simulink library "aerolib6dof2"  (Simulink 6.0)
settings: Solver=ode45  SolverMode=SingleTasking  StartTime=0.0  StopTime=10.0  RelTol=1e-3
values from neighbouring files (symbols this model uses):
  s = aeroliblist    [asbhelp.m]
undefined symbols (not defined in the file or in its folder): m
libraries: aerolib6dof2 x5, aerolib6dofsys x2, aerolibutil x2, aerolibconvert x2, simulink x1
settings Model: Creator=sgage  LastModifiedBy=sgage  ExtModeAutoUpdateStatusClock=off
settings DataIOCC: SignalLoggingName=logsOut
settings OptimizationCC: BooleanDataType=off
settings DebuggingCC: CheckExecutionContextPreStartOutputMsg=on  CheckExecutionContextRuntimeOutputMsg=on  SolverPrmCheckMsg=none
settings HardwareCC: TargetUnknown=on
settings GRTTargetCC: LifeSpan=inf
settings SFSimCC: SFSimApplyToAllLibs=on  SFSimBuildMode=Incremental

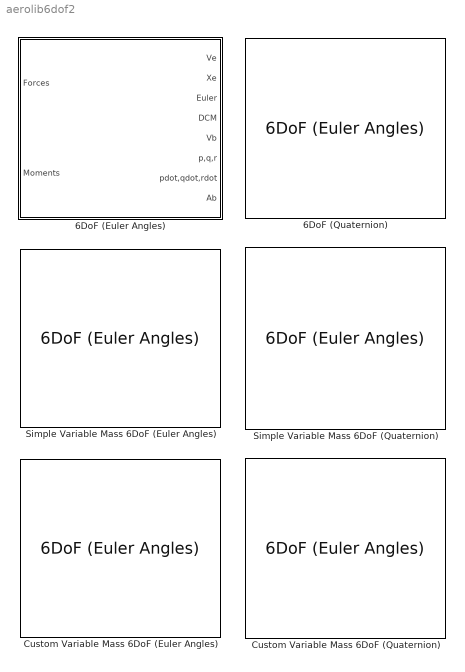
== system aerolib6dof2 ==
  6DoF (Euler Angles) : Subsystem  PropExecContextAcrossSSBoundary=on  mask(6DoF EoM (Body Axis)){units=Metric (MKS), mtype=Fixed, rep=Euler Angles, xme_0=[0 0 0], Vm_0=[0 0 0], eul_0=[0 0 0], pm_0=[0 0 0], mass_0=1.0, mass_e=0.5, mass_f=2.0, inertia=eye(3), inertia_e=eye(3), inertia_f=2*eye(3), k_quat=1.0}
      mask prompts: mtype "Mass type:"; rep "Representation:"; xme_0 "Initial position in inertial axes [Xe,Ye,Ze]:"; Vm_0 "Initial velocity in body axes [U,v,w]:"; eul_0 "Initial Euler orientation [roll, pitch, yaw]:"; pm_0 "Initial body rotation rates [p,q,r]:"; mass_0 "Initial mass:"; mass_e "Empty mass:"; mass_f "Full mass:"; inertia_e "Empty inertia matrix:"; inertia_f "Full inertia matrix:"; k_quat "Gain for quaternion normalization:"
      mask help: Integrate the six-degrees-of-freedom equations of motion using an Euler angle representation for the orientation of the body in space.
      mask init:
      | [x y xp yp highstr lowstr maxy miny]=aeroimage('sixdofbody');
      | ports=aeroicon('aeroblk6dofbody','icon');
      mask Help: web(asbhelp('6dofeulerangles'));
      mask StyleString: popup(Metric (MKS)|English (Velocity in ft/s)|English (Velocity in kts)),popup(Fixed|Simple Variable|Custom Variable),popup(Euler Angles|Quaternion),edit,edit,edit,edit,edit,edit,edit,edit,edit,edit,edit
      mask CallbackString: aeroicon('aeroblk6dofbody');|aeroicon('aeroblk6dofbody');|aeroicon('aeroblk6dofbody');|||||||||||
      mask Display:
      | port_label(ports(1).type,ports(1).port,ports(1).txt,'texmode','on');
      | port_label(ports(2).type,ports(2).port,ports(2).txt,'texmode','on');
      | port_label(ports(3).type,ports(3).port,ports(3).txt,'texmode','on');
      | port_label(ports(4).type,ports(4).port,ports(4).txt,'texmode','on');
      | port_label(ports(5).type,ports(5).port,ports(5).txt,'texmode','on');
      | port_label(ports(6).type,ports(6).port,ports(6).txt,'texmode','on');
      | port_label(ports(7).type,ports(7).port,ports(7).txt,'texmode','on');
      | port_label(ports(8).type,ports(8).port,ports(8).txt,'texmode','on');
      | port_label(ports(9).type,ports(9).port,ports(9).txt,'texmode','on');
      | port_label(ports(10).type,ports(10).port,ports(10).txt,'texmode','on');
      | port_label(ports(11).type,ports(11).port,ports(11).txt,'texmode','on');
      | port_label(ports(12).type,ports(12).port,ports(12).txt,'texmode','on');
      | port_label(ports(13).type,ports(13).port,ports(13).txt,'texmode','on');
      | port_label(ports(14).type,ports(14).port,ports(14).txt,'texmode','on');
      | port_label(ports(15).type,ports(15).port,ports(15).txt,'texmode','on');
      | text(0.5,maxy+0.05,highstr{:},'horizontalAlignment','center')
      | text(0.5,miny-0.05,lowstr{:},'horizontalAlignment','center')
      | plot(x,y);
      | patch(xp, yp);
  6DoF (Quaternion) : aerolib6dof2/6DoF (Euler Angles)  units=Metric (MKS)  mtype=Fixed  rep=Quaternion  xme_0=[0 0 0]  Vm_0=[0 0 0]  eul_0=[0 0 0]  pm_0=[0 0 0]  mass_0=1.0  mass_e=0  mass_f=0  inertia=eye(3)  inertia_e=eye(3)  inertia_f=eye(3)  k_quat=1.0
  Custom Variable Mass 6DoF (Euler Angles) : aerolib6dof2/6DoF (Euler Angles)  units=Metric (MKS)  mtype=Custom Variable  rep=Euler Angles  xme_0=[0 0 0]  Vm_0=[0 0 0]  eul_0=[0 0 0]  pm_0=[0 0 0]  mass_0=1.0  mass_e=0  mass_f=0  inertia=eye(3)  inertia_e=eye(3)  inertia_f=eye(3)  k_quat=1.0
  Custom Variable Mass 6DoF (Quaternion) : aerolib6dof2/6DoF (Euler Angles)  units=Metric (MKS)  mtype=Custom Variable  rep=Quaternion  xme_0=[0 0 0]  Vm_0=[0 0 0]  eul_0=[0 0 0]  pm_0=[0 0 0]  mass_0=1.0  mass_e=0  mass_f=0  inertia=eye(3)  inertia_e=eye(3)  inertia_f=eye(3)  k_quat=1.0
  Simple Variable Mass 6DoF (Euler Angles) : aerolib6dof2/6DoF (Euler Angles)  units=Metric (MKS)  mtype=Simple Variable  rep=Euler Angles  xme_0=[0 0 0]  Vm_0=[0 0 0]  eul_0=[0 0 0]  pm_0=[0 0 0]  mass_0=1.0  mass_e=0.5  mass_f=2.0  inertia=eye(3)  inertia_e=eye(3)  inertia_f=2*eye(3)  k_quat=1.0
  Simple Variable Mass 6DoF (Quaternion) : aerolib6dof2/6DoF (Euler Angles)  units=Metric (MKS)  mtype=Simple Variable  rep=Quaternion  xme_0=[0 0 0]  Vm_0=[0 0 0]  eul_0=[0 0 0]  pm_0=[0 0 0]  mass_0=1.0  mass_e=0.5  mass_f=2.0  inertia=eye(3)  inertia_e=eye(3)  inertia_f=2*eye(3)  k_quat=1.0

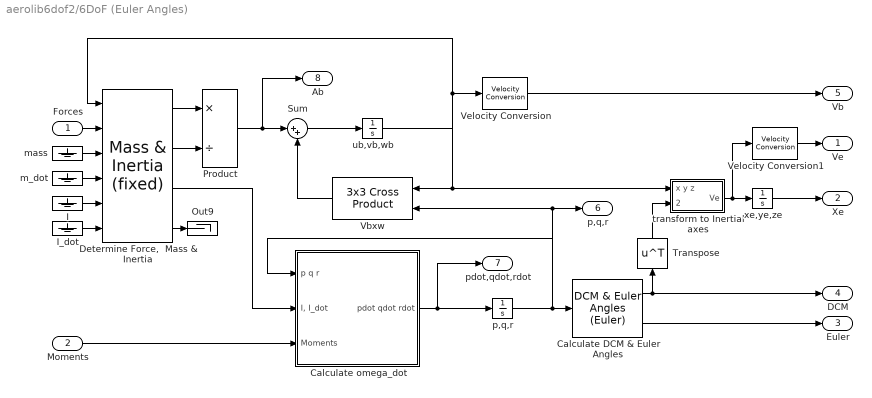
== system aerolib6dof2/6DoF (Euler Angles) ==
  Forces : Inport  LatchInput=off
  Moments : Inport  Port=2  LatchInput=off
  Calculate DCM & Euler Angles : aerolib6dofsys/DCM & Euler Angles (Euler)
  Calculate omega_dot : Subsystem  PropExecContextAcrossSSBoundary=on
  "Determine Force,  Mass & Inertia" : aerolib6dofsys/Mass & Inertia (fixed)
  I : Ground
  I_dot : Ground
  Out9 : Terminator
  Product : Product  Inputs=*/  SaturateOnIntegerOverflow=on
  Sum : Sum  Inputs=|++  SaturateOnIntegerOverflow=on
  Transpose : Math  Orientation=up  Operator=transpose  SaturateOnIntegerOverflow=on
  Vbxw : aerolibutil/3x3 Cross Product  Orientation=left
  Velocity Conversion : aerolibconvert/Velocity Conversion  IU=m/s  OU=m/s
  Velocity Conversion1 : aerolibconvert/Velocity Conversion  IU=m/s  OU=m/s
  m_dot : Ground
  mass : Ground
  "p,q,r " : Integrator  InitialCondition=pm_0
  "transform to Inertial axes " : Subsystem  PropExecContextAcrossSSBoundary=on
      mask Type: Vector Transformation
      mask Display: disp('L_EB')
  ub,vb,wb : Integrator  InitialCondition=Vm_0
  xe,ye,ze : Integrator  InitialCondition=xme_0
  Ve : Outport
  Xe : Outport  Port=2
  Euler : Outport  Port=3
  DCM : Outport  Port=4
  Vb : Outport  Port=5
  p,q,r : Outport  Port=6
  pdot,qdot,rdot : Outport  Port=7
  Ab : Outport  Port=8
  wires:
  Velocity Conversion1/1 -> Ve/1
  Velocity Conversion/1 -> Vb/1
  "Determine Force,  Mass & Inertia"/3 -> Calculate omega_dot/2("I, I_dot")
  Calculate DCM & Euler Angles/2 -> Euler/1
  Vbxw/1 -> Sum/2
  ub,vb,wb/1 -> Velocity Conversion/1, "transform to Inertial axes "/1(x y z), Vbxw/1, "Determine Force,  Mass & Inertia"/1
  Sum/1 -> ub,vb,wb/1
  xe,ye,ze/1 -> Xe/1
  "transform to Inertial axes "/1(Ve) -> Velocity Conversion1/1, xe,ye,ze/1
  "p,q,r "/1 -> p,q,r/1, Vbxw/2, Calculate omega_dot/1(p q r), Calculate DCM & Euler Angles/1
  Moments/1 -> Calculate omega_dot/3(Moments)
  Forces/1 -> "Determine Force,  Mass & Inertia"/2
  Product/1 -> Sum/1, Ab/1
  Calculate DCM & Euler Angles/1 -> DCM/1, Transpose/1
  Transpose/1 -> "transform to Inertial axes "/2(transform coefficients)
  mass/1 -> "Determine Force,  Mass & Inertia"/3
  "Determine Force,  Mass & Inertia"/2 -> Product/2
  m_dot/1 -> "Determine Force,  Mass & Inertia"/4
  "Determine Force,  Mass & Inertia"/4 -> Out9/1
  Calculate omega_dot/1(pdot qdot rdot) -> pdot,qdot,rdot/1, "p,q,r "/1
  I/1 -> "Determine Force,  Mass & Inertia"/5
  I_dot/1 -> "Determine Force,  Mass & Inertia"/6
  "Determine Force,  Mass & Inertia"/1 -> Product/1

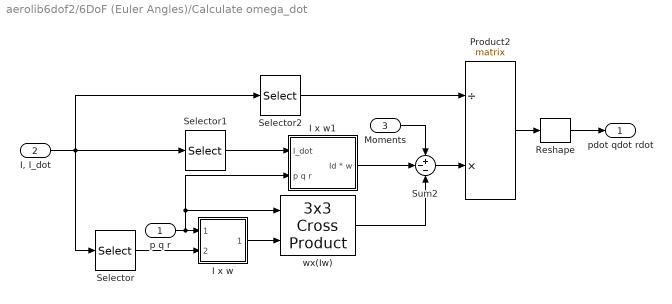
== system aerolib6dof2/6DoF (Euler Angles)/Calculate omega_dot ==
  p q r : Inport  LatchInput=off
  "I, I_dot" : Inport  Port=2  LatchInput=off
  Moments : Inport  Port=3  LatchInput=off
  I x w : Subsystem  PropExecContextAcrossSSBoundary=on
  I x w1 : Subsystem  PropExecContextAcrossSSBoundary=on
  Product2 : Product  Inputs=/*  Multiplication=Matrix(*)  SaturateOnIntegerOverflow=on
  Reshape : simulink/Math Operations/Reshape  OutputDimensionality=1-D array  OutputDimensions=[1,1]
  Selector : Selector  InputType=Matrix  Elements=[1 2 1]  Rows=1:3  Columns=-1  InputPortWidth=2
  Selector1 : Selector  InputType=Matrix  Elements=[1 2 1]  Rows=4:6  Columns=-1  InputPortWidth=2
  Selector2 : Selector  InputType=Matrix  Elements=[1 2 1]  Rows=1:3  Columns=-1  InputPortWidth=2
  Sum2 : Sum  Inputs=+--  SaturateOnIntegerOverflow=on
  wx(Iw) : aerolibutil/3x3 Cross Product
  pdot qdot rdot : Outport
  wires:
  I x w/1(I * w) -> wx(Iw)/2
  wx(Iw)/1 -> Sum2/3
  Selector1/1 -> I x w1/1(I_dot)
  I x w1/1(Id * w) -> Sum2/2
  Moments/1 -> Sum2/1
  Sum2/1 -> Product2/2
  Product2/1 -> Reshape/1
  p q r/1 -> I x w1/2(p q r), wx(Iw)/1, I x w/1(p q r)
  "I, I_dot"/1 -> Selector1/1, Selector2/1, Selector/1
  Selector2/1 -> Product2/1
  Selector/1 -> I x w/2(Inertia)
  Reshape/1 -> pdot qdot rdot/1

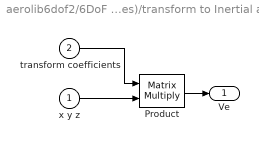
== system aerolib6dof2/6DoF (Euler Angles)/transform to Inertial axes  ==
  x y z : Inport  LatchInput=off
  transform coefficients : Inport  Port=2  LatchInput=off
  Product : Product  Multiplication=Matrix(*)  SaturateOnIntegerOverflow=on  InputSameDT=on
  Ve : Outport
  wires:
  Product/1 -> Ve/1
  transform coefficients/1 -> Product/1
  x y z/1 -> Product/2

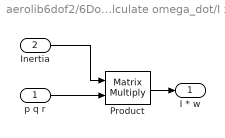
== system aerolib6dof2/6DoF (Euler Angles)/Calculate omega_dot/I x w ==
  p q r : Inport  LatchInput=off
  Inertia : Inport  Port=2  LatchInput=off
  Product : Product  Multiplication=Matrix(*)  SaturateOnIntegerOverflow=on  InputSameDT=on
  I * w : Outport
  wires:
  p q r/1 -> Product/2
  Inertia/1 -> Product/1
  Product/1 -> I * w/1

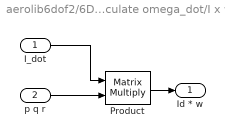
== system aerolib6dof2/6DoF (Euler Angles)/Calculate omega_dot/I x w1 ==
  I_dot : Inport  LatchInput=off
  p q r : Inport  Port=2  LatchInput=off
  Product : Product  Multiplication=Matrix(*)  SaturateOnIntegerOverflow=on  InputSameDT=on
  Id * w : Outport
  wires:
  Product/1 -> Id * w/1
  I_dot/1 -> Product/1
  p q r/1 -> Product/2
